simulink model "spiBitbangSimulink"  (R2013b)
settings: Solver=FixedStepDiscrete  StartTime=0.0  StopTime=5e-3  FixedStep=sampleTime  MaxStep=MaxStepSize  RelTol=1e-3
undefined symbols (not defined in the file or in its folder): periSam, pulseSam, sampleTime, sigbuilder_block
libraries: simulink x4, embdlinuxlib x2, dspswit3 x1, simulink_extras x1, dspsigops x1
settings Model: ExtModeTrigDuration=100  Creator=mainster  LastModifiedBy=mainster
settings OptimizationCC: OptimizeModelRefInitCode=on  LifeSpan=1
settings DebuggingCC: SolverPrmCheckMsg=none
settings HardwareCC: ProdLargestAtomicInteger=Long  ProdLargestAtomicFloat=Double  ProdEndianess=LittleEndian  ProdHWDeviceType=ARM Compatible->ARM Cortex
settings RTWCC: SystemTargetFile=realtime.tlc  GenerateMakefile=off  TemplateMakefile=realtime.tmf  Description=Run on Target Hardware  RTWVerbose=off  ProcessScript=realtime_make_rtw_hook
settings STFCustomTargetCC: TargetLibSuffix=.a  GenerateSampleERTMain=on  ERTCustomFileBanners=on  SupportNonInlinedSFcns=off  SupportVariableSizeSignals=on  MATLABClassNameForMDSCustomization=Simulink.SoftwareTarget.ERTCustomization  GRTInterface=off  SystemTargetFile=realtime.tlc
settings ERTTargetCC: CodeReplacementLibrary=ANSI_C  GenerateSampleERTMain=on  ParMdlRefBuildCompliant=off  CompOptLevelCompliant=off  ConcurrentExecutionCompliant=off  CombineOutputUpdateFcns=off  ERTFirstTimeCompliant=off  SupportContinuousTime=on  SupportVariableSizeSignals=on  ModelStepFunctionPrototypeControlCompliant=off  CPPClassGenCompliant=off  ExtModeMexArgs='192.168.2.111' 0 17725  InlinedParameterPlacement=NonHierarchical  ERTSrcFileBannerTemplate=realtime_code_template.cgt  ERTHdrFileBannerTemplate=realtime_code_template.cgt  ERTDataSrcFileTemplate=realtime_code_template.cgt  ERTDataHdrFileTemplate=realtime_code_template.cgt  ERTCustomFileTemplate=realtime_file_process.tlc

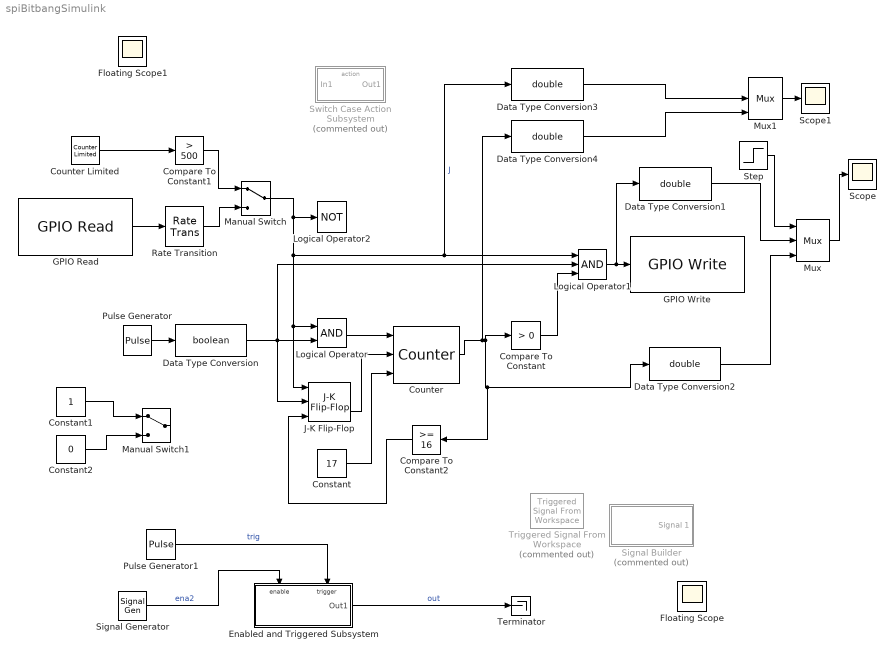
== system spiBitbangSimulink ==
  Compare To Constant : simulink/Logic and Bit Operations/Compare To Constant  relop=>  const=0  OutDataTypeStr=boolean
  Compare To Constant1 : simulink/Logic and Bit Operations/Compare To Constant  relop=>  const=500  OutDataTypeStr=boolean
  Compare To Constant2 : simulink/Logic and Bit Operations/Compare To Constant  relop=>=  const=16  OutDataTypeStr=boolean
  Constant : Constant  Value=17  OutDataTypeStr=uint8  LockScale=on
  Constant1 : Constant  OutDataTypeStr=boolean  SampleTime=-1
  Constant2 : Constant  Value=0  OutDataTypeStr=boolean  SampleTime=-1
  Counter : dspswit3/Counter  Direction=Up  CountEvent=Rising edge  CounterSize=Specify via input port  MaxCount=255  InitialCount=0  Output=Count  HitValue=2  ResetInput=on  SamplesPerFrame=1  Ts=1  CntDtype=uint8  HitDtype=Logical
  Counter Limited : simulink/Sources/Counter Limited  uplimit=800  tsamp=-1
  Data Type Conversion : DataTypeConversion  OutDataTypeStr=boolean  SampleTime=sampleTime
  Data Type Conversion{1..4} (4 alike) : DataTypeConversion  OutDataTypeStr=double  SampleTime=sampleTime
  Enabled and Triggered Subsystem : Subsystem  TreatAsAtomicUnit=on
  Floating Scope : Scope  NumInputPorts=3
      settings: Floating=on  TimeRange=0.006  YMin=-0.2~-5~-5  YMax=1.2~5~5  SaveName=ScopeData2
  GPIO Read : embdlinuxlib/GPIO Read  board=Model B Rev2  gpio=7  internalResistor=Off  sampleTime=sampleTimeGPIOin  direction=Input  blockPlatform=Raspberry Pi
  GPIO Write : embdlinuxlib/GPIO Write  board=Model B Rev2  gpio=15  direction=Output  blockPlatform=Raspberry Pi
  J-K Flip-Flop : simulink_extras/Flip Flops/J-K Flip-Flop  initial_condition=0
  Logical Operator : Logic  AllPortsSameDT=off  OutDataTypeStr=boolean
  Logical Operator1 : Logic  Inputs=3  AllPortsSameDT=off  OutDataTypeStr=boolean
  Logical Operator2 : Logic  Operator=NOT  Inputs=3  AllPortsSameDT=off  OutDataTypeStr=boolean
  Manual Switch : ManualSwitch
  Manual Switch1 : ManualSwitch
  Mux : Mux  Inputs=3
      settings: DisplayOption=signals
  Mux1 : Mux  Inputs=3
      settings: DisplayOption=signals
  Pulse Generator : DiscretePulseGenerator  Period=10  PulseWidth=5  SampleTime=-1
  Pulse Generator1 : DiscretePulseGenerator  Period=200  PulseWidth=150  SampleTime=sampleTime
  Rate Transition : RateTransition
  Scope : Scope
      settings: TimeRange=0.006000000000000005  YMin=-0.1  YMax=1.2
  Scope1 : Scope
      settings: TimeRange=0.006000000000000005  YMin=-1  YMax=17
  Signal Generator : SignalGenerator  WaveForm=square  Frequency=1e3
  Signal Builder : Subsystem  Tag=STV Subsys  Commented=on  LoadFcn=sigbuilder_block('load');  StartFcn=sigbuilder_block('start');  StopFcn=sigbuilder_block('stop');  ClipboardFcn=sigbuilder_block('clipboard');  mask(Sigbuilder block){}
      mask help: Simulink:masks:SigbuilderBlock_MD
      mask init:
      | if ~strcmp(get_param(bdroot(gcbh),'SimulationStatus'),'stopped') tuvar = sigbuilder_block('maskInit'); end
      settings: CopyFcn=sigbuilder_block('copy');  DeleteFcn=sigbuilder_block('delete');  ModelCloseFcn=sigbuilder_block('modelClose');  PreSaveFcn=sigbuilder_block('preSave');  PauseFcn=sigbuilder_block('pause');  ContinueFcn=sigbuilder_block('continue');  NameChangeFcn=sigbuilder_block('namechange');  OpenFcn=sigbuilder_block('open',[437.25 199.5 550.5 399.75 ]);  CloseFcn=sigbuilder_block('close');
      mask Display: plot(0, 0, 100, 100,[2, 2, 32, 32, 2], [68, 8, 8, 68, 68],[32, 2], [38, 38], [32, 19, 2],[53, 60, 44], [32, 17, 17, 2],[16, 16, 31, 31]);txt = getActiveGroup(gcbh);text(2, 100, txt,'verticalAlignment', 'top');
  Step : Step  Time=100*sampleTime  Before=-0.2  After=1.2
  Switch Case Action Subsystem : Subsystem  Commented=on  TreatAsAtomicUnit=on
  Terminator : Terminator
  Triggered Signal From Workspace : dspsigops/Triggered Signal From Workspace  Commented=on  Signal=1:10  TriggerType=Falling edge  ic=0  SamplesPerFrame=1  OutputAfterFinalValue=Setting to zero
  Floating Scope1 : Scope
      settings: Floating=on  SaveName=ScopeData3
  wires:
  GPIO Read/1 -> Rate Transition/1
  Data Type Conversion/1 -> J-K Flip-Flop/2, Logical Operator/2, Logical Operator1/2
  Pulse Generator/1 -> Data Type Conversion/1
  Logical Operator/1 -> Counter/1
  Counter/1 -> Data Type Conversion4/1, Compare To Constant2/1, Data Type Conversion2/1, Compare To Constant/1
  Logical Operator1/1 -> Data Type Conversion1/1, GPIO Write/1
  Compare To Constant/1 -> Logical Operator1/3
  Compare To Constant1/1 -> Manual Switch/1
  Step/1 -> Mux/1
  Mux/1 -> Scope/1
  Counter Limited/1 -> Compare To Constant1/1
  Rate Transition/1 -> Manual Switch/2
  Data Type Conversion1/1 -> Mux/2
  Manual Switch/1 -> Logical Operator2/1, Data Type Conversion3/1, Logical Operator1/1, J-K Flip-Flop/1, Logical Operator/1  "J"
  Data Type Conversion2/1 -> Mux/3
  Mux1/1 -> Scope1/1
  Data Type Conversion3/1 -> Mux1/2
  Data Type Conversion4/1 -> Mux1/3
  Constant/1 -> Counter/3
  Compare To Constant2/1 -> J-K Flip-Flop/3
  J-K Flip-Flop/2 -> Counter/2
  Constant1/1 -> Manual Switch1/1
  Constant2/1 -> Manual Switch1/2
  Enabled and Triggered Subsystem/1(Out1) -> Terminator/1  "out"
  Pulse Generator1/1 -> Enabled and Triggered Subsystem/Trigger  "trig"
  Signal Generator/1 -> Enabled and Triggered Subsystem/Enable  "ena2"

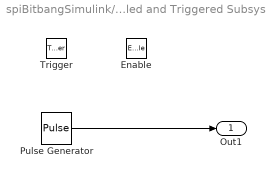
== system spiBitbangSimulink/Enabled and Triggered Subsystem ==
  Enable : EnablePort
  Trigger : TriggerPort
  Pulse Generator : DiscretePulseGenerator  Period=periSam  PulseWidth=pulseSam  SampleTime=-1
  Out1 : Outport
  wires:
  Pulse Generator/1 -> Out1/1

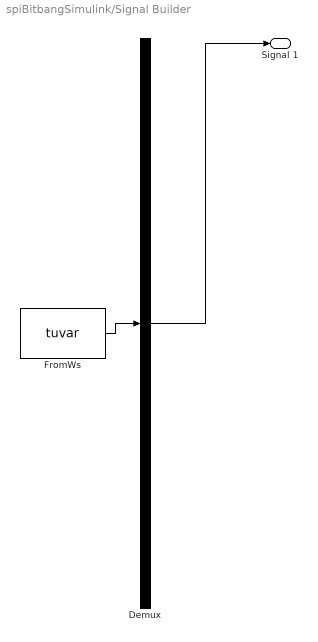
== system spiBitbangSimulink/Signal Builder ==
  Demux : Demux  Tag=STV Demux  Outputs=1
  FromWs : FromWorkspace  Tag=STV FromWs  VariableName=tuvar  SampleTime=0
      SigBuilderData=|
      | common.afterFinalStr = 'Extrapolate'
      | common.sampleTime = 0
      | dataSet.timeRange = [0 10]
      | dataSet.name = 'Group 1'
      | sbobj.Groups.Name = 'Group 1'
      | sbobj.Groups.Signals.Name = 'Signal 1'
      | sbobj.Groups.Signals.XData = [0 4 4 6 6 10]
      | sbobj.Groups.Signals.YData = [0 0 1 1 0 0]
  Signal 1 : Outport  Tag=STV Outport
  wires:
  Demux/1 -> Signal 1/1
  FromWs/1 -> Demux/1

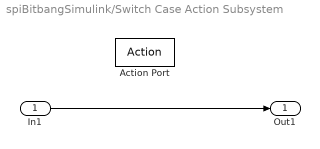
== system spiBitbangSimulink/Switch Case Action Subsystem ==
  In1 : Inport
  Action Port : ActionPort
  Out1 : Outport
  wires:
  In1/1 -> Out1/1
